simulink model "simu_complete"  (R2024b)
settings: Solver=FixedStepAuto  StartTime=0.0  StopTime=Tsim  FixedStep=Ts  RelTol=1e-3
values from neighbouring files (symbols this model uses):
  Tr = 0.5    [main_phi.m]
undefined symbols (not defined in the file or in its folder): delta0, deltaF, Re, t_sw, v0
settings Model: Creator=marti  LastModifiedBy=Filip

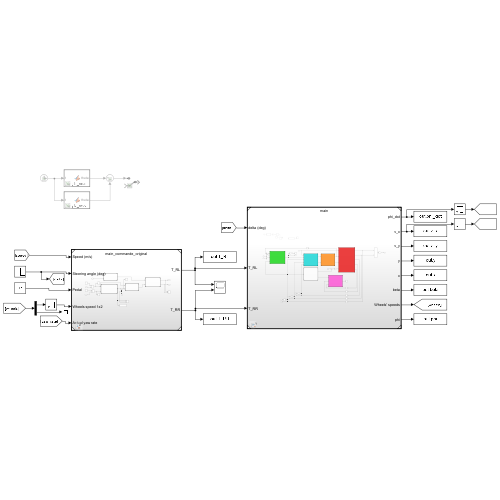
[thumbnail: Simulink's stored preview of the top-level diagram]
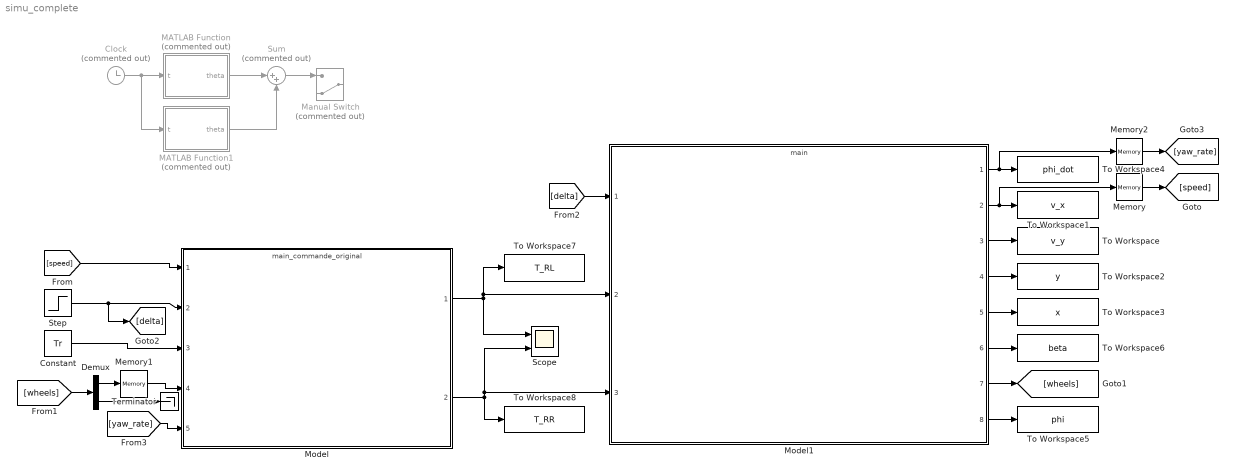
== system simu_complete ==
  Clock : Clock  Commented=on
  Constant : Constant  Value=Tr
  Demux : Demux  Outputs=2
  MATLAB Function : MATLAB Function  Commented=on  TreatAsAtomicUnit=on
  MATLAB Function1 : MATLAB Function  Commented=on  TreatAsAtomicUnit=on
  Manual Switch : ManualSwitch  Commented=on  CurrentSetting=0
  Memory : Memory  InitialCondition=v0
  Memory1 : Memory  InitialCondition=[v0/Re v0/Re]
  Memory2 : Memory
  Model : ModelReference  ModelNameDialog=main_commande_original.slx  SimulationMode=Normal  ModelReferenceVersion=1.29
  Model1 : ModelReference  ModelNameDialog=main.slx  SimulationMode=Normal  ModelReferenceVersion=1.137
  Scope : Scope  NumInputPorts=2
  Step : Step  Time=t_sw  Before=delta0  After=deltaF  SampleTime=0
  Sum : Sum  Commented=on  Inputs=|++
  Terminator : Terminator
  To Workspace : ToWorkspace  VariableName=v_y  SaveFormat=Structure With Time  SampleTime=-1
  To Workspace1 : ToWorkspace  VariableName=v_x  SaveFormat=Structure With Time  SampleTime=-1
  To Workspace2 : ToWorkspace  VariableName=y  SaveFormat=Structure With Time  SampleTime=-1
  To Workspace3 : ToWorkspace  VariableName=x  SaveFormat=Structure With Time  SampleTime=-1
  To Workspace4 : ToWorkspace  VariableName=phi_dot  SaveFormat=Structure With Time  SampleTime=-1
  To Workspace5 : ToWorkspace  VariableName=phi  SaveFormat=Structure With Time  SampleTime=-1
  To Workspace6 : ToWorkspace  VariableName=beta  SaveFormat=Structure With Time  SampleTime=-1
  To Workspace7 : ToWorkspace  VariableName=T_RL  SaveFormat=Structure With Time  SampleTime=-1
  To Workspace8 : ToWorkspace  VariableName=T_RR  SaveFormat=Structure With Time  SampleTime=-1
  wires:
  Model1/2 -> To Workspace1/1, Memory/1
  [speed] -> Model/1
  [wheels] -> Demux/1
  Demux/1 -> Memory1/1
  Clock/1 -> MATLAB Function1/1(t), MATLAB Function/1(t)
  Constant/1 -> Model/3
  [delta] -> Model1/1
  Memory/1 -> [speed]
  Model1/7 -> [wheels]
  Memory1/1 -> Model/4
  Model1/1 -> To Workspace4/1, Memory2/1
  Memory2/1 -> [yaw_rate]
  Sum/1 -> Manual Switch/1
  Step/1 -> [delta], Model/2
  [yaw_rate] -> Model/5
  MATLAB Function/1(theta) -> Sum/1
  MATLAB Function1/1(theta) -> Sum/2
  Demux/2 -> Terminator/1
  Model1/8 -> To Workspace5/1
  Model1/3 -> To Workspace/1
  Model1/4 -> To Workspace2/1
  Model1/5 -> To Workspace3/1
  Model1/6 -> To Workspace6/1
  Model/1 -> To Workspace7/1, Model1/2, Scope/1
  Model/2 -> Scope/2, Model1/3, To Workspace8/1

== matlab function simu_complete/MATLAB Function ==
  data: t input; theta output
function theta = angle_roue(t)
    % Fonction pour modéliser l'angle de roue d'un double changement de voie
    % Entrée :
    %   t : vecteur ou scalaire temps
    % Sortie :
    %   theta : angle de roue correspondant à chaque t

    theta = zeros(size(t));  % Initialisation

    % Intervalle actif : [1,4]
    idx = (t > 1) & (t < 4);
    
    % Fonction sinus entre 2 et 5 (période complète sur 3 secondes)
    theta(idx) = sin(2*pi * (t(idx) - 1) / 3);
end

== matlab function simu_complete/MATLAB Function1 ==
  data: t input; theta output
function theta = angle_roue(t)
    % Fonction pour modéliser l'angle de roue d'un double changement de voie
    % Entrée :
    %   t : vecteur ou scalaire temps
    % Sortie :
    %   theta : angle de roue correspondant à chaque t

    theta = zeros(size(t));  % Initialisation

    % Intervalle actif : [5,8]
    idx = (t > 6) & (t < 9);
    
    % Fonction sinus entre 2 et 5 (période complète sur 3 secondes)
    theta(idx) = -sin(2*pi * (t(idx) - 6) / 3);
end
